simulink model "mtq_model_test"  (R2018b)
settings: Solver=VariableStepAuto  StartTime=0.0  StopTime=10.0  RelTol=1e-3
undefined symbols (not defined in the file or in its folder): fswParams
libraries: vrlib x2, mtq_model_lib x1, clock_lib x1, time_Lib x1, magField_lib x1, sgp4_lib_fsw x1
settings Model: Creator=taylorreynolds  LastModifiedBy=taylorreynolds

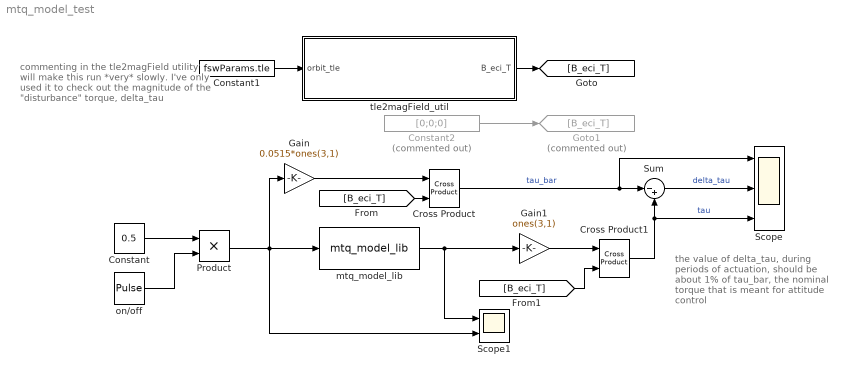
== system mtq_model_test ==
  note: the value of delta_tau, during
      | periods of actuation, should be
      | about 1% of tau_bar, the nominal
      | torque that is meant for attitude
      | control
  note: commenting in the tle2magField
      | utility will make this run *very*
      | slowly. I've only used it to check
      | out the magnitude of the "disturbance"
      | torque, delta_tau
  Constant : Constant  Value=0.5
  Constant1 : Constant  Value=fswParams.tle
  Constant2 : Constant  Commented=on  Value=[0;0;0]
  Cross Product : vrlib/Utilities/Cross Product
      settings: SourceProductBaseCode=VR
  Cross Product1 : vrlib/Utilities/Cross Product
      settings: SourceProductBaseCode=VR
  Gain : Gain  Gain=0.0515*ones(3,1)
  Gain1 : Gain  Gain=ones(3,1)
  Goto1 : Goto  Commented=on  GotoTag=B_eci_T
  Product : Product
  Scope : Scope  NumInputPorts=3
  Scope1 : Scope  NumInputPorts=2
  Sum : Sum  Inputs=|-+
  mtq_model_lib : mtq_model_lib/mtq_model_lib  R=23.2  L=0.15  Vs=5  Fsw=5000  NA=0.23896
  on/off : DiscretePulseGenerator  PulseType=Time based  PulseWidth=50
  tle2magField_util : Subsystem
  wires:
  Product/1 -> Scope1/2, mtq_model_lib/1, Gain/1
  on/off/1 -> Product/2
  mtq_model_lib/1 -> Scope1/1, Gain1/1
  Constant/1 -> Product/1
  Gain/1 -> Cross Product/1
  Constant1/1 -> tle2magField_util/1(orbit_tle)
  tle2magField_util/1(B_eci_T) -> [B_eci_T]
  [B_eci_T] -> Cross Product/2
  Cross Product/1 -> Scope/1, Sum/1  "tau_bar"
  [B_eci_T] -> Cross Product1/2
  Cross Product1/1 -> Scope/3, Sum/2  "tau"
  Sum/1 -> Scope/2  "delta_tau"
  Gain1/1 -> Cross Product1/1
  Constant2/1 -> Goto1/1

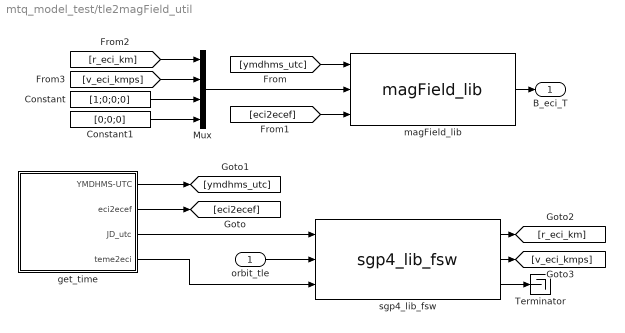
== system mtq_model_test/tle2magField_util ==
  orbit_tle : Inport
  Constant : Constant  Value=[1;0;0;0]
  Constant1 : Constant  Value=[0;0;0]
  Mux : Mux  Inputs=[3 3 4 3]
  Terminator : Terminator
  get_time : Subsystem
  magField_lib : magField_lib/magField_lib  SystemSampleTime=-1
  sgp4_lib_fsw : sgp4_lib_fsw/sgp4_lib_fsw  SystemSampleTime=-1
  B_eci_T : Outport
  wires:
  Constant1/1 -> Mux/4
  Constant/1 -> Mux/3
  [v_eci_kmps] -> Mux/2
  [r_eci_km] -> Mux/1
  sgp4_lib_fsw/2 -> [v_eci_kmps]
  sgp4_lib_fsw/1 -> [r_eci_km]
  [eci2ecef] -> magField_lib/3
  [ymdhms_utc] -> magField_lib/1
  orbit_tle/1 -> sgp4_lib_fsw/2
  get_time/4(teme2eci) -> sgp4_lib_fsw/3
  get_time/3(JD_utc) -> sgp4_lib_fsw/1
  sgp4_lib_fsw/3 -> Terminator/1
  magField_lib/1 -> B_eci_T/1
  get_time/1(YMDHMS-UTC) -> [ymdhms_utc]
  Mux/1 -> magField_lib/2
  get_time/2(eci2ecef) -> [eci2ecef]

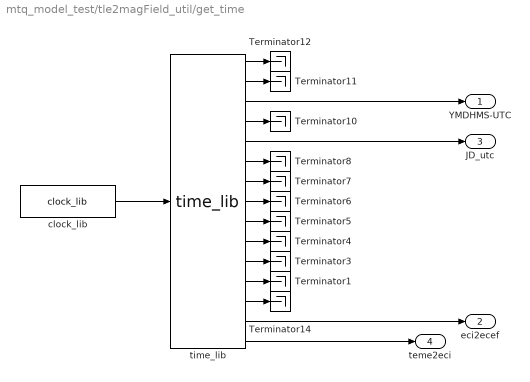
== system mtq_model_test/tle2magField_util/get_time ==
  Terminator{1,3..8,10..12,14} (11 alike) : Terminator
  clock_lib : clock_lib/clock_lib  SystemSampleTime=-1
  "time_lib " : time_Lib/time_lib    SystemSampleTime=-1
  YMDHMS-UTC : Outport
  eci2ecef : Outport  Port=2
  JD_utc : Outport  Port=3
  teme2eci : Outport  Port=4
  wires:
  "time_lib "/5 -> JD_utc/1
  "time_lib "/15 -> teme2eci/1
  "time_lib "/1 -> Terminator12/1
  "time_lib "/2 -> Terminator11/1
  "time_lib "/4 -> Terminator10/1
  "time_lib "/6 -> Terminator8/1
  "time_lib "/7 -> Terminator7/1
  "time_lib "/8 -> Terminator6/1
  "time_lib "/9 -> Terminator5/1
  "time_lib "/10 -> Terminator4/1
  "time_lib "/11 -> Terminator3/1
  "time_lib "/12 -> Terminator1/1
  "time_lib "/13 -> Terminator14/1
  "time_lib "/14 -> eci2ecef/1
  "time_lib "/3 -> YMDHMS-UTC/1
  clock_lib/1 -> "time_lib "/1
